simulink model "PB2M_001_007"  (R2024a)
settings: Solver=FixedStepDiscrete  StartTime=0.0  StopTime=24*366  FixedStep=[global_ST]  RelTol=1e-3
model workspace (MAT data in the model file):
  Var = 0
values from neighbouring files (symbols this model uses):
  global_ST = 1    [SimControl_v3_rl.m]    (also in SimControl_v4.m)
  global_time = [0:1:8784]'    [SimControl_v3_rl.m]    (also in SimControl_v4.m)
undefined symbols (not defined in the file or in its folder): AEL, AMB, ATR, Bttry, CGH2, CGO2, CHP, chp, COMPR, Ctrl, DiscIntNeverNeededParam, DIST, DRY, GASF, Gasf, MES, PV, th, WT
(part 2 of 2)

== matlab function PB2M_001_007/BM /MATLAB Function ==
  data: mflow_H2 input; module output; mflow_SG input; th parameter; ATR parameter
function module = module_calc(mflow_H2, mflow_SG, th, ATR)
module = module_calc_ex(mflow_H2, mflow_SG, th, ATR);

end

== matlab function PB2M_001_007/BM /Ideal Controller ==
  data: fac input; CHP input; Hydrogen input; GASF parameter; DRY parameter; ATR parameter; BM_wet output
function BM_wet = biopath(fac, CHP, Hydrogen, GASF, DRY, ATR)
BM_wet = biopath_ex(Hydrogen, fac, CHP, ATR, GASF, DRY);
end

== stateflow chart PB2M_001_007/O2 Distribution/O2_DISTRIBUTION ==
  state ACTION
    O2_req = SMR_req + GASF_req;
    shortage = O2_req - AEL_act;
    CGO2_maxIn = (CGO2_cap - CGO2_lvl) * 1000 / 720;
    CGO2_maxOut = CGO2_lvl * 1000 / 720;
    state Surplus
      CGO2_out = 0;
      CGO2_in = min(abs(shortage), CGO2_maxIn);
      SMR = SMR_req;
      GASF = GASF_req;
    state Shortage
      CGO2_out = min(shortage, CGO2_maxOut);
      CGO2_in = 0;
      SMR = SMR_req;
      GASF = GASF_req;
    (default) -> Shortage
    Shortage -> Surplus : [shortage <= 0]
    Surplus -> Shortage : [shortage > 0]
  data: SMR_req input; AEL_act input; CGO2_in output; CGO2_out output; SMR output; O2_req local; shortage local; CGO2_lvl input; CGO2_cap constant double =CGO2.Cap; CGO2_maxIn local; CGO2_maxOut local; GASF_req input; GASF output

== matlab function PB2M_001_007/WT, PV/PHOTOVOLTAIC/Panel Efficiency ==
  data: G input; eta output; t input; PV parameter
function eta = TotalEff(G, t, PV)

eta = PV_PanelEff_Ex(G, t, PV);

end

== matlab function PB2M_001_007/ctrl/MATLAB Function ==
  data: CHP output; Battery_in output; P_in input; P_sec input; Battery_lvl input; Battery_SOC input; CGH2_lvl input; CGH2_SOC input; Battery_out output; Grid output; P_prim output; curt output; Bttry parameter; CGH2 parameter; AEL parameter; Gasf parameter; CGH2_out output; CGH2_in output; OZ output; Ctrl parameter; chp parameter; rL output; Battery_maxIn output; Battery_maxOut output; CGH2_maxIn output; CGH2_maxOut output
function [CHP, Battery_in, Battery_out, Grid, P_prim, curt, CGH2_out, CGH2_in, OZ, rL, Battery_maxIn, Battery_maxOut, CGH2_maxIn, CGH2_maxOut] =    manage_power_v8(P_in, P_sec, Battery_lvl, Battery_SOC, CGH2_lvl, CGH2_SOC, Bttry, CGH2, AEL, Gasf, Ctrl, chp)

         [CHP, Battery_in, Battery_out, Grid, P_prim, curt, CGH2_out, CGH2_in, OZ, rL, Battery_maxIn, Battery_maxOut, CGH2_maxIn, CGH2_maxOut] = manage_power_ex_v8(P_in, P_sec, Battery_lvl, Battery_SOC, CGH2_lvl, CGH2_SOC, Bttry, CGH2, AEL, Gasf, Ctrl, chp);

end
